simulink model "doi_tuong_2022"  (R2022a)
settings: Solver=ode15s  StartTime=0.0  StopTime=50000  MaxStep=20000.0  RelTol=1e-3
undefined symbols (not defined in the file or in its folder): den_G11, den_G12, den_G21, den_G22, den_Gd1, den_Gd2, num_G11, num_G12, num_G21, num_G22, num_Gd1, num_Gd2
settings Model: Creator=PC  LastModifiedBy=Moderator
settings ModelReferenceCC: EnableRefExpFcnMdlSchedulingChecks=off
settings RTWCC: Description=Generic Real-Time Target  GPUComputeCapability=5.0

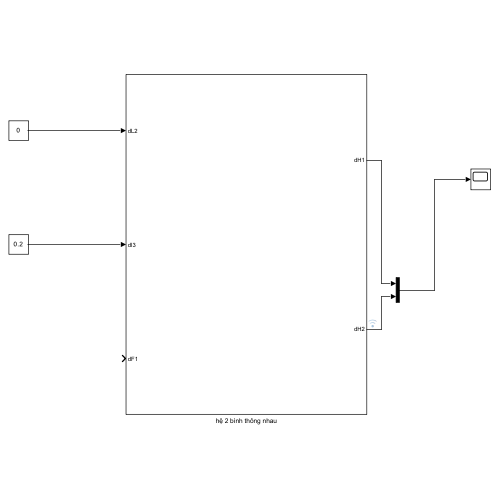
[thumbnail: Simulink's stored preview of the top-level diagram]
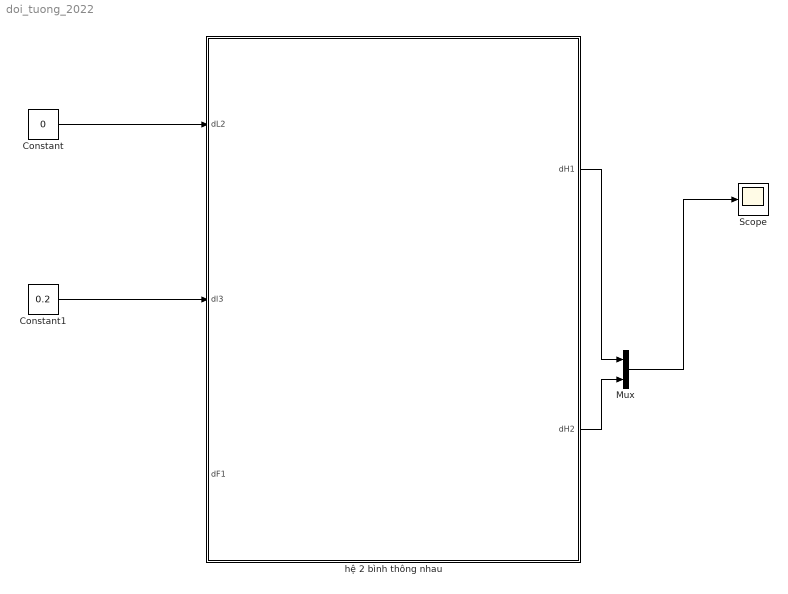
== system doi_tuong_2022 ==
  Constant : Constant  Value=0
  Constant1 : Constant  Value=0.2
  Mux : Mux  Inputs=2
  Scope : Scope
  hệ 2 bình thông nhau : Subsystem
  wires:
  Constant/1 -> hệ 2 bình thông nhau/1(dL2)
  Constant1/1 -> hệ 2 bình thông nhau/2(dl3)
  Mux/1 -> Scope/1
  hệ 2 bình thông nhau/1(dH1) -> Mux/1
  hệ 2 bình thông nhau/2(dH2) -> Mux/2

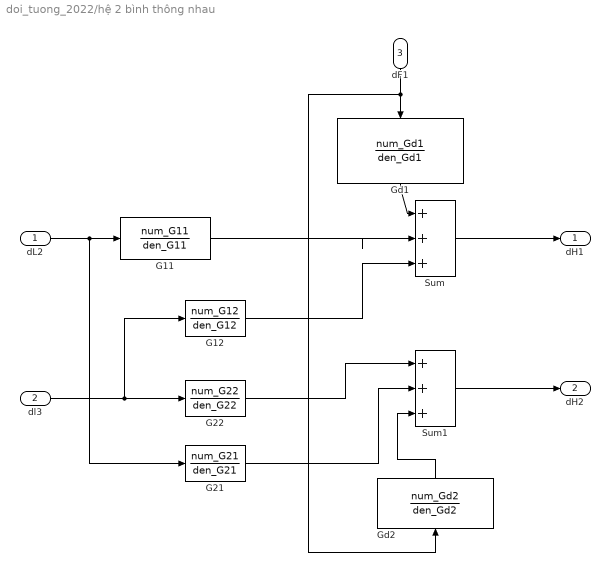
== system doi_tuong_2022/hệ 2 bình thông nhau ==
  dL2 : Inport
  dl3 : Inport  Port=2
  "dF1 " : Inport  Port=3
  G11 : TransferFcn  Numerator=num_G11  Denominator=den_G11
  G12 : TransferFcn  Numerator=num_G12  Denominator=den_G12
  G21 : TransferFcn  Numerator=num_G21  Denominator=den_G21
  G22 : TransferFcn  Numerator=num_G22  Denominator=den_G22
  Gd1 : TransferFcn  Numerator=num_Gd1  Denominator=den_Gd1
  Gd2 : TransferFcn  Numerator=num_Gd2  Denominator=den_Gd2
  Sum : Sum  Inputs=|+++
  Sum1 : Sum  Inputs=|+++
  dH1 : Outport
  dH2 : Outport  Port=2
  wires:
  G11/1 -> Sum/2
  G21/1 -> Sum1/2
  dl3/1 -> G12/1, G22/1
  dL2/1 -> G21/1, G11/1
  Gd1/1 -> Sum/1
  Gd2/1 -> Sum1/3
  G12/1 -> Sum/3
  "dF1 "/1 -> Gd2/1, Gd1/1
  Sum1/1 -> dH2/1
  Sum/1 -> dH1/1
  G22/1 -> Sum1/1
